simulink model "Problem_8"  (R2020a)
settings: Solver=VariableStepAuto  StartTime=0.0  StopTime=10.0  RelTol=1e-3
settings Model: Creator=Saqlain  LastModifiedBy=Saqlain

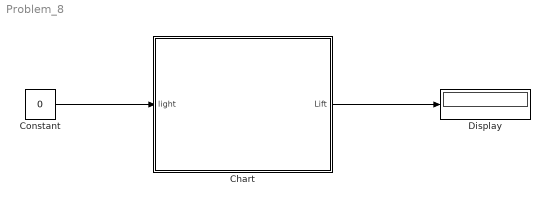
== system Problem_8 ==
  Chart : Stateflow chart  TreatAsAtomicUnit=on
  Constant : Constant  Value=0
  Display : Display
  wires:
  Chart/1(Lift) -> Display/1
  Constant/1 -> Chart/1(light)

== stateflow chart Problem_8/Chart ==
  state LIFT
    state LIFT_OFF
      en:
      Lift=0;
    state LIFT_ON
      en:
      Lift=1;
    (default) -> LIFT_OFF
    LIFT_OFF -> LIFT_ON : [light==1]
    LIFT_ON -> LIFT_OFF : [light==0]
  (default) -> LIFT
  data: Lift output; light input
